simulink model "timeDelay_SS"  (R2022a)
settings: Solver=VariableStepAuto  StartTime=0.0  StopTime=2  RelTol=1e-3
values from neighbouring files (symbols this model uses):
  Aaug = [Ad Bd;zeros(1,3) 0]    [ControllerwithDelay.m]    (also in ControllerwithDelay_LQR.m; ControllerwithDelay_SS.m; DiscreteObserver.m = Ad-Bd)
  Aaug2 = [Ad zeros(3,1) Bd; -Cd 1 0;zeros(1,5)]    [ControllerwithDelay_SS.m]
  Ad = ss_d.A    [ControllerwithDelay.m]    (also in ControllerwithDelay_LQR.m; ControllerwithDelay_PID.m; ControllerwithDelay_SS.m; DiscreteLQControl.m)
  Adaug = [Ad zeros(3,1);-Cd 1]    [ControllerwithDelay_SS.m]    (also in steadyStateError.m = [Ad zeros(size(Ad,1),1); Cd 1])
  Baug = [0;0;0;1]    [ControllerwithDelay.m]    (also in ControllerwithDelay_LQR.m; ControllerwithDelay_SS.m)
  Baug2 = [zeros(3,1);0;1]    [ControllerwithDelay_SS.m]
  Bd = ss_d.B    [ControllerwithDelay.m]    (also in ControllerwithDelay_LQR.m; ControllerwithDelay_PID.m; ControllerwithDelay_SS.m; DiscreteLQControl.m)
  Bdaug = [Bd; 0]    [ControllerwithDelay_SS.m]    (also in steadyStateError.m)
  Caug = [1 0 0 0]    [ControllerwithDelay.m]    (also in ControllerwithDelay_LQR.m; ControllerwithDelay_SS.m)
  Caug2 = [1 0 0 0 0]    [ControllerwithDelay_SS.m]
  Cd = ss_d.C    [ControllerwithDelay.m]    (also in ControllerwithDelay_LQR.m; ControllerwithDelay_PID.m; ControllerwithDelay_SS.m; DiscreteLQControl.m)
  Cdaug = [1 0 0 0]    [ControllerwithDelay_SS.m]    (also in steadyStateError.m = [Cd 0])
  kDisc_dr = place(Adaug,Bdaug,[0.2 0.2+0.1j 0.2-0.1j 0.8])    [ControllerwithDelay_SS.m]
  kDisc_dr2 = place(Aaug2,Baug2,[0.2 0.2+0.1j 0.2-0.1j 0.8 1])    [ControllerwithDelay_SS.m]
  kDisc_dr_delay = place(Aaug2,Baug2,[0.2 0.2+0.1j 0.2-0.1j 0.8 0.1])    [ControllerwithDelay_SS.m]
  kDisc_dr_delay2 = place(Aaug2,Baug2,[0.2 0.2+0.1j 0.2-0.1j 0.12 0.1])    [ControllerwithDelay_SS.m]
  kDisc_new = place(Aaug,Baug,[0.5 0.4+0.5j 0.4-0.5j 0.6])    [ControllerwithDelay_SS.m]
  kDisc_new2 = place(Aaug,Baug,[0.5 0.4+0.5j 0.4-0.5j 0.1])    [ControllerwithDelay_SS.m]
  kDisc_new3 = place(Aaug,Baug,[0.2 0.2+0.1j 0.2-0.1j 0.1])    [ControllerwithDelay_SS.m]
  kDisc_old = place(Ad,Bd,[0.5 0.4+0.5j 0.4-0.5j])    [ControllerwithDelay_SS.m]
  kDisc_old2 = place(Aaug,Baug,[0.5 0.4+0.5j 0.4-0.5j 1.1])    [ControllerwithDelay_SS.m]
settings Model: Creator=1  LastModifiedBy=1

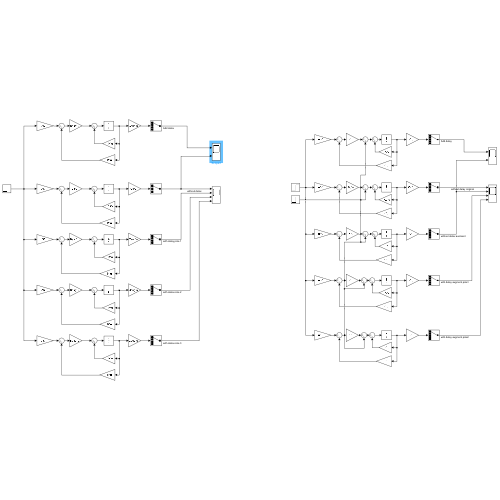
[thumbnail: Simulink's stored preview of the top-level diagram]
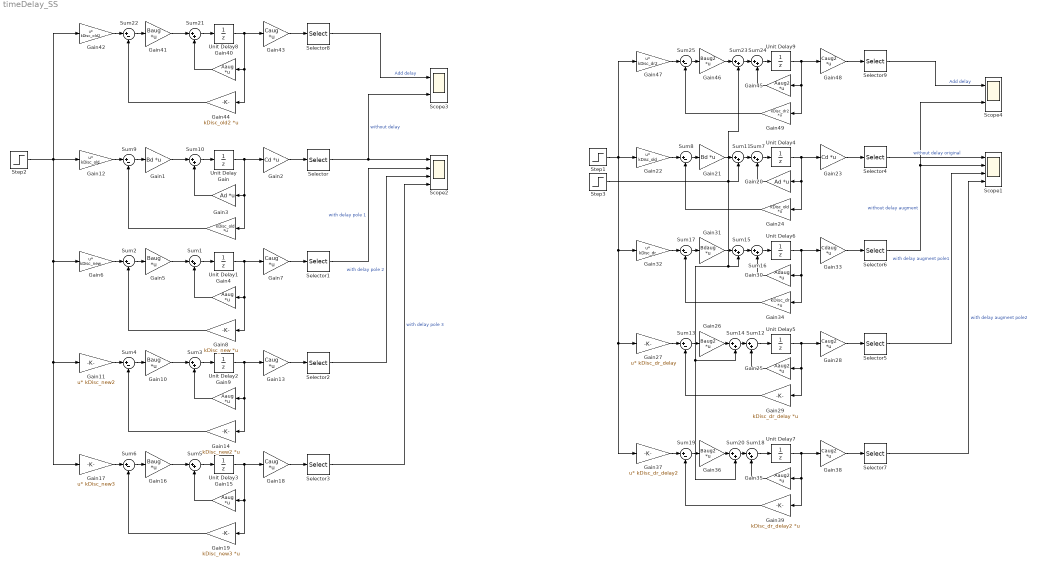
== system timeDelay_SS ==
  Gain : Gain  Gain=Ad  Multiplication=Matrix(K*u)
  Gain1 : Gain  Gain=Bd  Multiplication=Matrix(K*u)
  Gain{5,10,16,41} (4 alike) : Gain  Gain=Baug  Multiplication=Matrix(K*u)
  Gain11 : Gain  Gain=kDisc_new2  Multiplication=Matrix(u*K)
  Gain12 : Gain  Gain=kDisc_old  Multiplication=Matrix(u*K)
  Gain{7,13,18,43} (4 alike) : Gain  Gain=Caug  Multiplication=Matrix(K*u)
  Gain14 : Gain  Gain=kDisc_new2  Multiplication=Matrix(K*u)
  Gain{4,9,15,40} (4 alike) : Gain  Gain=Aaug  Multiplication=Matrix(K*u)
  Gain17 : Gain  Gain=kDisc_new3  Multiplication=Matrix(u*K)
  Gain19 : Gain  Gain=kDisc_new3  Multiplication=Matrix(K*u)
  Gain2 : Gain  Gain=Cd  Multiplication=Matrix(K*u)
  Gain20 : Gain  Gain=Ad  Multiplication=Matrix(K*u)
  Gain21 : Gain  Gain=Bd  Multiplication=Matrix(K*u)
  Gain22 : Gain  Gain=kDisc_old  Multiplication=Matrix(u*K)
  Gain23 : Gain  Gain=Cd  Multiplication=Matrix(K*u)
  Gain24 : Gain  Gain=kDisc_old  Multiplication=Matrix(K*u)
  Gain25 : Gain  Gain=Aaug2  Multiplication=Matrix(K*u)
  Gain26 : Gain  Gain=Baug2  Multiplication=Matrix(K*u)
  Gain27 : Gain  Gain=kDisc_dr_delay  Multiplication=Matrix(u*K)
  Gain28 : Gain  Gain=Caug2  Multiplication=Matrix(K*u)
  Gain29 : Gain  Gain=kDisc_dr_delay  Multiplication=Matrix(K*u)
  Gain3 : Gain  Gain=kDisc_old  Multiplication=Matrix(K*u)
  Gain30 : Gain  Gain=Adaug  Multiplication=Matrix(K*u)
  Gain31 : Gain  Gain=Bdaug  Multiplication=Matrix(K*u)
  Gain32 : Gain  Gain=kDisc_dr  Multiplication=Matrix(u*K)
  Gain33 : Gain  Gain=Cdaug  Multiplication=Matrix(K*u)
  Gain34 : Gain  Gain=kDisc_dr  Multiplication=Matrix(K*u)
  Gain35 : Gain  Gain=Aaug2  Multiplication=Matrix(K*u)
  Gain36 : Gain  Gain=Baug2  Multiplication=Matrix(K*u)
  Gain37 : Gain  Gain=kDisc_dr_delay2  Multiplication=Matrix(u*K)
  Gain38 : Gain  Gain=Caug2  Multiplication=Matrix(K*u)
  Gain39 : Gain  Gain=kDisc_dr_delay2  Multiplication=Matrix(K*u)
  Gain42 : Gain  Gain=kDisc_old2  Multiplication=Matrix(u*K)
  Gain44 : Gain  Gain=kDisc_old2  Multiplication=Matrix(K*u)
  Gain45 : Gain  Gain=Aaug2  Multiplication=Matrix(K*u)
  Gain46 : Gain  Gain=Baug2  Multiplication=Matrix(K*u)
  Gain47 : Gain  Gain=kDisc_dr2  Multiplication=Matrix(u*K)
  Gain48 : Gain  Gain=Caug2  Multiplication=Matrix(K*u)
  Gain49 : Gain  Gain=kDisc_dr2  Multiplication=Matrix(K*u)
  Gain6 : Gain  Gain=kDisc_new  Multiplication=Matrix(u*K)
  Gain8 : Gain  Gain=kDisc_new  Multiplication=Matrix(K*u)
  Scope1 : Scope  NumInputPorts=4
  Scope2 : Scope  NumInputPorts=4
  Scope3 : Scope  NumInputPorts=2
  Scope4 : Scope  NumInputPorts=2
  Selector : Selector  InputPortWidth=3  IndexOptions=Index vector (dialog)  Indices=[1]  OutputSizes=1
  Selector{1..3,6,8} (5 alike) : Selector  InputPortWidth=4  IndexOptions=Index vector (dialog)  Indices=[1]  OutputSizes=1
  Selector4 : Selector  InputPortWidth=3  IndexOptions=Index vector (dialog)  Indices=[1]  OutputSizes=1
  Selector5 : Selector  InputPortWidth=5  IndexOptions=Index vector (dialog)  Indices=[1]  OutputSizes=1
  Selector7 : Selector  InputPortWidth=5  IndexOptions=Index vector (dialog)  Indices=[1]  OutputSizes=1
  Selector9 : Selector  InputPortWidth=5  IndexOptions=Index vector (dialog)  Indices=[1]  OutputSizes=1
  Step1 : Step  Time=0.1  After=0  SampleTime=0
  Step2 : Step  Time=0.1  SampleTime=0
  Step3 : Step  Time=0.1  SampleTime=0
  Sum{1,3,5,7,10..12,14..16,18,20..21,23..24} (15 alike) : Sum  Inputs=|++
  Sum{2,4,6,8..9,13,17,19,22,25} (10 alike) : Sum  Inputs=|+-
  Unit Delay{,1..9} (10 alike) : UnitDelay  SampleTime=-1  HasFrameUpgradeWarning=on
  wires:
  Gain12/1 -> Sum9/1
  Selector/1 -> Scope3/2, Scope2/1  "without delay"
  Gain2/1 -> Selector/1
  Gain3/1 -> Sum9/2
  Sum9/1 -> Gain1/1
  Unit Delay/1 -> Gain3/1, Gain/1, Gain2/1
  Gain1/1 -> Sum10/1
  Gain/1 -> Sum10/2
  Sum10/1 -> Unit Delay/1
  Step2/1 -> Gain42/1, Gain17/1, Gain11/1, Gain6/1, Gain12/1
  Sum2/1 -> Gain5/1
  Gain8/1 -> Sum2/2
  Sum1/1 -> Unit Delay1/1
  Gain5/1 -> Sum1/1
  Gain4/1 -> Sum1/2
  Gain6/1 -> Sum2/1
  Unit Delay1/1 -> Gain8/1, Gain4/1, Gain7/1
  Gain7/1 -> Selector1/1
  Selector1/1 -> Scope2/2  "with delay pole 1"
  Unit Delay2/1 -> Gain14/1, Gain9/1, Gain13/1
  Gain13/1 -> Selector2/1
  Gain11/1 -> Sum4/1
  Gain14/1 -> Sum4/2
  Gain9/1 -> Sum3/2
  Gain10/1 -> Sum3/1
  Sum3/1 -> Unit Delay2/1
  Sum4/1 -> Gain10/1
  Unit Delay3/1 -> Gain19/1, Gain15/1, Gain18/1
  Gain18/1 -> Selector3/1
  Gain17/1 -> Sum6/1
  Gain19/1 -> Sum6/2
  Gain15/1 -> Sum5/2
  Gain16/1 -> Sum5/1
  Sum5/1 -> Unit Delay3/1
  Sum6/1 -> Gain16/1
  Selector2/1 -> Scope2/3  "with delay pole 2"
  Selector3/1 -> Scope2/4  "with delay pole 3"
  Sum8/1 -> Gain21/1
  Selector4/1 -> Scope1/1  "without delay original"
  Gain24/1 -> Sum8/2
  Gain23/1 -> Selector4/1
  Sum7/1 -> Unit Delay4/1
  Gain22/1 -> Sum8/1
  Unit Delay4/1 -> Gain24/1, Gain20/1, Gain23/1
  Gain20/1 -> Sum7/2
  Step1/1 -> Gain47/1, Gain32/1, Gain37/1, Gain27/1, Gain22/1
  Gain21/1 -> Sum11/1
  Sum11/1 -> Sum7/1
  Step3/1 -> Sum23/2, Sum15/2, Sum20/2, Sum14/2, Sum11/2
  Unit Delay5/1 -> Gain29/1, Gain25/1, Gain28/1
  Gain28/1 -> Selector5/1
  Gain27/1 -> Sum13/1
  Gain29/1 -> Sum13/2
  Gain25/1 -> Sum12/2
  Sum12/1 -> Unit Delay5/1
  Sum13/1 -> Gain26/1
  Gain26/1 -> Sum14/1
  Sum14/1 -> Sum12/1
  Selector5/1 -> Scope1/3  "with delay augment pole1"
  Gain31/1 -> Sum15/1
  Gain30/1 -> Sum16/2
  Unit Delay6/1 -> Gain34/1, Gain30/1, Gain33/1
  Gain33/1 -> Selector6/1
  Sum17/1 -> Gain31/1
  Gain34/1 -> Sum17/2
  Sum15/1 -> Sum16/1
  Sum16/1 -> Unit Delay6/1
  Gain32/1 -> Sum17/1
  Selector6/1 -> Scope4/2, Scope1/2  "without delay augment"
  Sum20/1 -> Sum18/1
  Unit Delay7/1 -> Gain39/1, Gain35/1, Gain38/1
  Gain36/1 -> Sum20/1
  Gain38/1 -> Selector7/1
  Sum19/1 -> Gain36/1
  Sum18/1 -> Unit Delay7/1
  Gain35/1 -> Sum18/2
  Gain39/1 -> Sum19/2
  Gain37/1 -> Sum19/1
  Selector7/1 -> Scope1/4  "with delay augment pole2"
  Unit Delay8/1 -> Gain44/1, Gain40/1, Gain43/1
  Gain43/1 -> Selector8/1
  Gain42/1 -> Sum22/1
  Gain44/1 -> Sum22/2
  Gain40/1 -> Sum21/2
  Gain41/1 -> Sum21/1
  Sum21/1 -> Unit Delay8/1
  Sum22/1 -> Gain41/1
  Selector8/1 -> Scope3/1  "Add delay"
  Gain47/1 -> Sum25/1
  Sum25/1 -> Gain46/1
  Sum24/1 -> Unit Delay9/1
  Sum23/1 -> Sum24/1
  Gain48/1 -> Selector9/1
  Unit Delay9/1 -> Gain49/1, Gain45/1, Gain48/1
  Gain46/1 -> Sum23/1
  Gain45/1 -> Sum24/2
  Gain49/1 -> Sum25/2
  Selector9/1 -> Scope4/1  "Add delay"
